simulink model "Testbench_ReferencePointCalculation"  (R2017b)
settings: Solver=VariableStepAuto  StartTime=0.0  StopTime=10.0  RelTol=1e-3
libraries: Lib_ReferencePointCalculation x1
settings Model: Creator=bernhard  LastModifiedBy=esterle

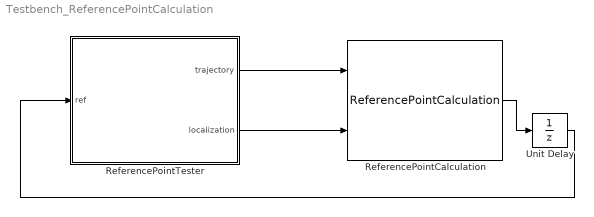
== system Testbench_ReferencePointCalculation ==
  ReferencePointCalculation : Lib_ReferencePointCalculation/ReferencePointCalculation
  "ReferencePointTester " : MATLAB Function  TreatAsAtomicUnit=on
  Unit Delay : UnitDelay  SampleTime=-1
  wires:
  "ReferencePointTester "/1(trajectory) -> ReferencePointCalculation/1
  "ReferencePointTester "/2(localization) -> ReferencePointCalculation/2
  ReferencePointCalculation/1 -> Unit Delay/1
  Unit Delay/1 -> "ReferencePointTester "/1(ref)

== matlab function Testbench_ReferencePointCalculation/ReferencePointTester  ==
  data: trajectory output Bus: ControlTrajectory; ref input Bus: TrajectoryPoint; localization output Bus: LocalizationToAutobox
function [trajectory, localization]  = ReferencePointTester(ref)
coder.extrinsic('display')
persistent test_number;

num_points = 1000;

trajectory = struct('n_trajectory_point',uint32(0),...
    'x',zeros(num_points,1), ...
    'y',zeros(num_points,1), ...
    'z', zeros(num_points,1), ...
    'theta', zeros(num_points,1), ...
    'kappa',zeros(num_points,1), ...
    'dkappa', zeros(num_points,1), ...
    'ddkappa', zeros(num_points,1), ...
    's', zeros(num_points,1), ...
    'v', zeros(num_points,1), ...
    'a', zeros(num_points,1), ...
    'relative_time',zeros(num_points,1), ...
    'timestamp_sec', zeros(1,1));

point3d = struct('x',double(0),'y', double(0),'z',double(0));
point_enu= struct('x', double(0),'y', double(0),'z',double(0));
quaternion = struct('qx', double(0),'qy',double(0),'qz',double(0),'qw',double(0));

pose = struct('Position', point_enu, ...
    'Orientation',quaternion,...
    'LinearVelocity',point3d, ...
    'LinearAcceleration',point3d, ...
    'AngularVelocity',point3d, ...
    'Heading',double(0),...
    'LinearAccelerationVrf',point3d, ...
    'AngularVelocityVrf',point3d, ...
    'EulerAngles',point3d);

uncertainty = struct('PositionStdDev',point3d, ...
    'OrientationStdDev',point3d,...
    'LinearVelocityStdDev',point3d, ...
    'LinearAccelerationStdDev',point3d, ...
    'AngularVelocityStdDev',point3d);

localization  = struct('Pose', pose, 'MeasurementTime', double(0), 'Uncertainty', uncertainty);

if isempty(test_number)
    test_number=0;
end


if test_number == 0
    %Zeroth Test: Linear Position Change from x=10 to x=99m in 100 seconds,
    %timestamp 5s
    trajectory.x = linspace(0,99,num_points)';
    trajectory.y = zeros(num_points,1);
    trajectory.z = zeros(num_points,1);
    trajectory.theta = zeros(num_points,1);
    trajectory.kappa = zeros(num_points,1);
    trajectory.dkappa = zeros(num_points,1);
    trajectory.ddkappa = zeros(num_points,1);
    trajectory.s = zeros(num_points,1);
    trajectory.v = zeros(num_points,1);
    trajectory.a = zeros(num_points,1);
    trajectory.relative_time = linspace(0,99,num_points)';
    trajectory.timestamp_sec = 5;
    trajectory.n_trajectory_point=uint32(num_points);
    
    localization.MeasurementTime = 9.5;
    
    test_number = test_number + 1;
elseif test_number == 1
    % check previous outcome
    if ref.x ~= 4.5 % absolute timestamp = 5, measurement time = 9.5
        display("ERROR in test 0: ref.x ~= 4.5");
    else
        display("Test 0 success.");
    end
    
    %First Test: Linear Position Change from x=10 to x=num_pointsm and y=0m to
    %99m in 100 seconds, timestamp 20s, should take last point exactly
    trajectory.x = linspace(0,99,num_points)';
    trajectory.y = linspace(0,99,num_points)';
    trajectory.z = zeros(num_points,1);
    trajectory.theta = zeros(num_points,1);
    trajectory.kappa = zeros(num_points,1);
    trajectory.dkappa = zeros(num_points,1);
    trajectory.ddkappa = zeros(num_points,1);
    trajectory.s = zeros(num_points,1);
    trajectory.v = zeros(num_points,1);
    trajectory.a = zeros(num_points,1);
    trajectory.relative_time = linspace(0,99,num_points)';
    trajectory.timestamp_sec = 20;
    trajectory.n_trajectory_point=uint32(num_points);
    
    localization.MeasurementTime = 119; % this should be last point in trajectory
    
    test_number = test_number +1;
elseif test_number == 2
    % check previous outcome
    if ref.x ~= 99 && ref.y ~= 99
        display("ERROR in test 1: ref.x ~= 99 && ref.y ~= 99");
    else
        display("Test 1 success.");
    end
    % Second Test, only one valid trajectory point given, with measurement
    % time larger than point time
    trajectory.x = linspace(1,100,num_points)';
    trajectory.y = zeros(num_points,1);
    trajectory.z = zeros(num_points,1);
    trajectory.theta = zeros(num_points,1);
    trajectory.kappa = zeros(num_points,1);
    trajectory.dkappa = zeros(num_points,1);
    trajectory.ddkappa = zeros(num_points,1);
    trajectory.s = zeros(num_points,1);
    trajectory.v = zeros(num_points,1);
    trajectory.a = zeros(num_points,1);
    trajectory.relative_time = linspace(1,100,num_points)';
    trajectory.relative_time(2:end) = 0; % test if num max points 10 is correctly considered
    trajectory.timestamp_sec = 0;
    trajectory.n_trajectory_point=uint32(1);
    
    localization.MeasurementTime = 1.1;
    
    
    test_number = test_number +1;
    
elseif test_number == 3
    % check previous outcome
    if ref.x ~= 1
        display("ERROR in test 2: ref.x ~= 1");
    else
        display("Test 2 success.");
    end
    
    % Third Test, only one valid trajectory point given, with exact matching on this
    % trajectory point
    trajectory.x = linspace(1,100,num_points)';
    trajectory.y = zeros(num_points,1);
    trajectory.z = zeros(num_points,1);
    trajectory.theta = zeros(num_points,1);
    trajectory.kappa = zeros(num_points,1);
    trajectory.dkappa = zeros(num_points,1);
    trajectory.ddkappa = zeros(num_points,1);
    trajectory.s = zeros(num_points,1);
    trajectory.v = zeros(num_points,1);
    trajectory.a = zeros(num_points,1);
    trajectory.relative_time = linspace(1,100,num_points)';
    trajectory.relative_time(2:end) = 0; % test if num max points 10 is correctly considered
    trajectory.timestamp_sec = 0;
    trajectory.n_trajectory_point=uint32(1);
    
    localization.MeasurementTime = 1;
    
    
    test_number = test_number +1;
    
elseif test_number == 4
    % check previous outcome
    if ref.x ~= 1
        display("ERROR in test 3: ref.x ~= 1");
    else
        display("Test 3 success.");
    end
    
    % Fourth Test, , only two valid trajectory points given, non-integer
    % absoulute timestamp
    trajectory.x = linspace(1,100,num_points)';
    trajectory.y = zeros(num_points,1);
    trajectory.z = zeros(num_points,1);
    trajectory.theta = zeros(num_points,1);
    trajectory.kappa = zeros(num_points,1);
    trajectory.dkappa = zeros(num_points,1);
    trajectory.ddkappa = zeros(num_points,1);
    trajectory.s = zeros(num_points,1);
    trajectory.v = zeros(num_points,1);
    trajectory.a = zeros(num_points,1);
    trajectory.relative_time = linspace(1,100,num_points)';
    trajectory.relative_time(3:end) = 0; % test if num max points 10 is correctly considered
    trajectory.timestamp_sec = 0.5;
    trajectory.n_trajectory_point=uint32(2);
    
    localization.MeasurementTime = 2;
    
    test_number = test_number +1;
    
elseif test_number == 5
    % check previous outcome
    if ref.x ~= 1.5
        display("ERROR in test 4: ref.x ~= 2");
    else
        display("Test 4 success.");
    end
    
    % Fifth Test, interpolate orientation correctly
    trajectory.x = zeros(num_points,1);
    trajectory.y = zeros(num_points,1);
    trajectory.z = zeros(num_points,1);
    trajectory.theta = zeros(num_points,1);
    trajectory.theta(1) = 0.1;
    trajectory.theta(2) = -0.1;
    trajectory.kappa = zeros(num_points,1);
    trajectory.dkappa = zeros(num_points,1);
    trajectory.ddkappa = zeros(num_points,1);
    trajectory.s = zeros(num_points,1);
    trajectory.v = zeros(num_points,1);
    trajectory.a = zeros(num_points,1);
    trajectory.relative_time = linspace(0,99,num_points)';
    trajectory.relative_time(3:end) = 0; % test if num max points 10 is correctly considered
    trajectory.timestamp_sec = 0;
    trajectory.n_trajectory_point=uint32(2);
    
    localization.MeasurementTime = 0.5;
    
    test_number = test_number +1;
    
elseif test_number == 6
    
    if ref.theta ~= 0.0
        display("ERROR in test 5: ref.theta ~= 0.0");
    else
        display("Test 5 success.");
    end
    
    % Sixth Test, interpolate orientation correctly
    trajectory.x = zeros(num_points,1);
    trajectory.y = zeros(num_points,1);
    trajectory.z = zeros(num_points,1);
    trajectory.theta = zeros(num_points,1);
    trajectory.theta(1) = 0.1;
    trajectory.theta(2) = 2*pi-0.1;
    trajectory.kappa = zeros(num_points,1);
    trajectory.dkappa = zeros(num_points,1);
    trajectory.ddkappa = zeros(num_points,1);
    trajectory.s = zeros(num_points,1);
    trajectory.v = zeros(num_points,1);
    trajectory.a = zeros(num_points,1);
    trajectory.relative_time = linspace(0,99,num_points)';
    trajectory.relative_time(3:end) = 0; % test if num max points 10 is correctly considered
    trajectory.timestamp_sec = 0;
    trajectory.n_trajectory_point=uint32(2);
    
    localization.MeasurementTime = 0.5;
    
    test_number = test_number +1;
elseif test_number == 7
    if abs(ref.theta) > 0.00000001
        display("ERROR in test 6: abs(ref.theta) > 0.00000001");
    else
        display("Test 6 success.");
    end
    
    % Seventh Test, interpolate orientation correctly
    trajectory.x = zeros(num_points,1);
    trajectory.y = zeros(num_points,1);
    trajectory.z = zeros(num_points,1);
    trajectory.theta = zeros(num_points,1);
    trajectory.theta(1) = 2*pi-0.1;
    trajectory.theta(2) = 2*pi-0.3;
    trajectory.kappa = zeros(num_points,1);
    trajectory.dkappa = zeros(num_points,1);
    trajectory.ddkappa = zeros(num_points,1);
    trajectory.s = zeros(num_points,1);
    trajectory.v = zeros(num_points,1);
    trajectory.a = zeros(num_points,1);
    trajectory.relative_time = linspace(0,99,num_points)';
    trajectory.relative_time(3:end) = 0; % test if num max points 10 is correctly considered
    trajectory.timestamp_sec = 0;
    trajectory.n_trajectory_point=uint32(2);
    
    localization.MeasurementTime = 0.5;
    
    test_number = test_number +1;
    
elseif test_number == 8
    if ref.theta > -0.2 + 0.00000001 || ref.theta < -0.2 - 0.00000001
        display("ERROR in test 7: ref.theta ~= -0.2");
    else
        display("Test 7 success.");
    end
    
else
    % send default trajectory
    trajectory.x = linspace(1,100,num_points)';
    trajectory.y = zeros(num_points,1);
    trajectory.z = zeros(num_points,1);
    trajectory.theta = zeros(num_points,1);
    trajectory.kappa = zeros(num_points,1);
    trajectory.dkappa = zeros(num_points,1);
    trajectory.ddkappa = zeros(num_points,1);
    trajectory.s = zeros(num_points,1);
    trajectory.v = zeros(num_points,1);
    trajectory.a = zeros(num_points,1);
    trajectory.relative_time = linspace(1,100,num_points)';
    trajectory.timestamp_sec = 25.5;
    trajectory.n_trajectory_point=uint32(56);
    
    localization.MeasurementTime =10;
    
end
